simulink model "gm_transmitter"  (R2020b)
settings: Solver=FixedStepDiscrete  StartTime=0.0  StopTime=100000  RelTol=1e-3
undefined symbols (not defined in the file or in its folder): message
libraries: hdlmdlgenlib x28, simulink x10, hdlsllib x9, dspsigops x8, dspmlti4 x2, whdlio x1
(part 1 of 2)
settings Model: Creator=wardo  LastModifiedBy=wardo
settings DataIOCC: LimitDataPoints=on  SaveOutput=off  SaveTime=off
settings OptimizationCC: BlockReduction=off  ConditionallyExecuteInputs=off  DefaultParameterBehavior=Inlined  LifeSpan=inf
settings DebuggingCC: AlgebraicLoopMsg=error  InheritedTsInSrcMsg=none  SingleTaskRateTransMsg=error  AllowSymbolicDim=off  StrictBusMsg=ErrorOnBusTreatedAsVector  SFUnexpectedBacktrackingDiag=warning  SFNoUnconditionalDefaultTransitionDiag=warning  SFExecutionAtInitializationDiag=none  ArithmeticOperatorsInVariantConditions=warning
settings HardwareCC: ProdBitPerPointer=32  ProdBitPerSizeT=32  ProdBitPerPtrDiffT=32  ProdLargestAtomicFloat=None  ProdIntDivRoundTo=Undefined  ProdEndianess=Unspecified  ProdWordSize=32  ProdHWDeviceType=ASIC/FPGA->ASIC/FPGA  ProdEqTarget=off
settings SFSimCC: SimUseLocalCustomCode=off  CustomCodeUndefinedFunction=UseInterfaceOnly
settings RTWCC: RTWUseLocalCustomCode=off
settings CodeAppCC: StateflowObjectComments=on
settings GRTTargetCC: TargetLangStandard=C89/C90 (ANSI)
settings ConfigComp: CovScope=ReferencedModels  CovMetricSettings=dw  CovSaveCumulativeToWorkspaceVar=on  CovSaveSingleToWorkspaceVar=on  CovExternalEMLEnable=off  CovSFcnEnable=off

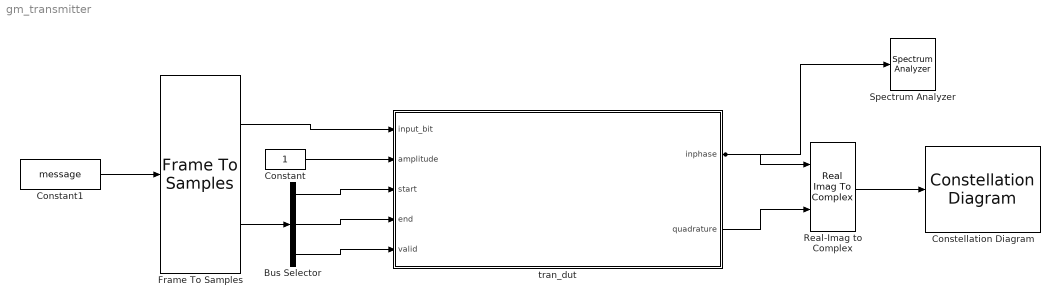
== system gm_transmitter ==
  Bus Selector : BusSelector  OutputSignals=start,end,valid
  Constant : Constant  OutDataTypeStr=uint8  SampleTime=-1
  Constant1 : Constant  Value=message  OutDataTypeStr=fixdt(0,1,0)  SampleTime=100000
  Constellation Diagram : ConstellationDiagram
  Frame To Samples : whdlio/Frame To Samples  InterSampleIdleCycles=0  InterFrameIdleCycles=0  OutputSize=1  InterleaveSamples=off
      settings: SourceProductBaseCode=LH
  Real-Imag to Complex : RealImagToComplex
  Spectrum Analyzer : SpectrumAnalyzer
  tran_dut : Subsystem
  wires:
  Bus Selector/3 -> tran_dut/5(valid)
  Bus Selector/2 -> tran_dut/4(end)
  Bus Selector/1 -> tran_dut/3(start)
  Frame To Samples/2 -> Bus Selector/1
  tran_dut/2(quadrature) -> Real-Imag to Complex/2
  tran_dut/1(inphase) -> Real-Imag to Complex/1, Spectrum Analyzer/1
  Real-Imag to Complex/1 -> Constellation Diagram/1
  Constant1/1 -> Frame To Samples/1
  Constant/1 -> tran_dut/2(amplitude)
  Frame To Samples/1 -> tran_dut/1(input_bit)

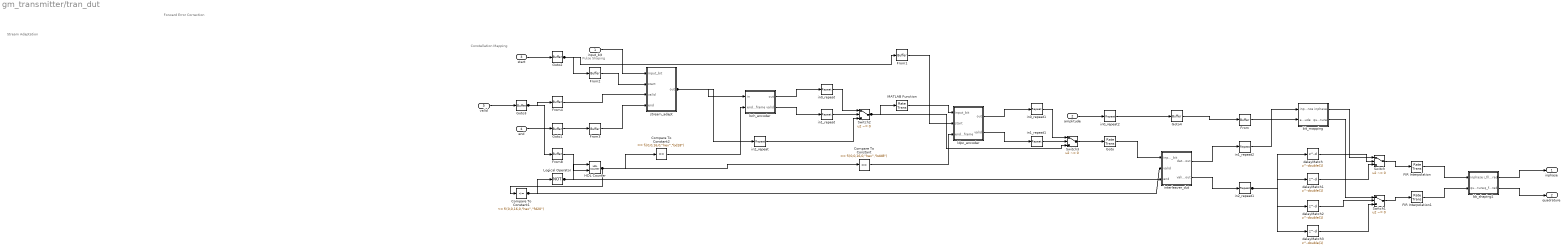
== system gm_transmitter/tran_dut ==
  note: Stream Adaptation
  note: Forward Error Correction
  note: Constellation Mapping
  note: Pulse Shaping
  input_bit : Inport  OutDataTypeStr=fixdt(0, 1, 0)  PortDimensions=1  SampleTime=2.06577425218972
  amplitude : Inport  Port=2  OutDataTypeStr=uint8  PortDimensions=1  SampleTime=2.06577425218972
  start : Inport  Port=3  OutDataTypeStr=boolean  PortDimensions=1  SampleTime=2.06577425218972
  end : Inport  Port=4  OutDataTypeStr=boolean  PortDimensions=1  SampleTime=2.06577425218972
  valid : Inport  Port=5  OutDataTypeStr=boolean  PortDimensions=1  SampleTime=2.06577425218972
  Compare To Constant : simulink/Logic and Bit Operations/Compare To Constant  relop===  const="fi(0,0,16,0,\"hex\",\"bdd8\")"  OutDataTypeStr=boolean
  Compare To Constant1 : simulink/Logic and Bit Operations/Compare To Constant  relop=<=  const="fi(0,0,16,0,\"hex\",\"fd20\")"  OutDataTypeStr=boolean
  Compare To Constant2 : simulink/Logic and Bit Operations/Compare To Constant  relop===  const="fi(0,0,16,0,\"hex\",\"bd18\")"  OutDataTypeStr=boolean
  FIR Interpolation : RateTransition  OutPortSampleTimeOpt=Multiple of input port sample time  OutPortSampleTimeMultiple=8
  FIR Interpolation1 : RateTransition  OutPortSampleTimeOpt=Multiple of input port sample time  OutPortSampleTimeMultiple=8
  From{,1..4,8} (6 alike) : hdlmdlgenlib/Buffer
      settings: SourceProductBaseCode=SL
  Goto : RateTransition  OutPortSampleTimeOpt=Multiple of input port sample time  OutPortSampleTimeMultiple=8
  Goto{1..4} (4 alike) : hdlmdlgenlib/Buffer
      settings: SourceProductBaseCode=SL
  HDL Counter : hdlsllib/Sources/HDL Counter  CountType=Count limited  CountInit=double(0)  CountStep=double(1)  CountMax=double(64800)  CountFromType=Initial value  CountFrom=double(0)  CountResetPort=on  CountLoadPort=off  CountEnbPort=on  CountDirPort=off  CountDataType=Unsigned  CountWordLen=16  CountFracLen=0  CountSampTime=2.06577425218972
  Logical Operator : Logic  Operator=NOT  Inputs=1  AllPortsSameDT=off  OutDataTypeStr=boolean  SampleTime=2.06577425218972
  MATLAB Function : RateTransition  OutPortSampleTimeOpt=Multiple of input port sample time  OutPortSampleTimeMultiple=8
  Switch : Switch  Criteria=u2 ~= 0  Threshold=double(0)  OutDataTypeStr=fixdt(1, 25, 15)  SampleTime=0.258221781523715
  Switch1 : Switch  Criteria=u2 ~= 0  Threshold=double(0)  OutDataTypeStr=fixdt(1, 25, 15)  SampleTime=0.258221781523715
  Switch2 : Switch  Criteria=u2 ~= 0  Threshold=double(0)  OutDataTypeStr=boolean  SampleTime=0.258221781523715
  Switch3 : Switch  Criteria=u2 ~= 0  Threshold=double(0)  OutDataTypeStr=boolean  SampleTime=0.258221781523715
  bb_shaping1 : Subsystem
  bch_encoder : Subsystem
  bit_mapping : Subsystem
  delayMatch{,1..3} (4 alike) : Delay  DelayLength=double(1)  InitialCondition=0  SampleTime=0.258221781523715
  in0_repeat : dspsigops/Repeat  N=double(8)  RateOptions=Allow multirate processing  ic=0  mode=Unused parameter value
  in0_repeat1 : dspsigops/Repeat  N=double(8)  RateOptions=Allow multirate processing  ic=0  mode=Unused parameter value
  in0_repeat2 : dspsigops/Repeat  N=double(8)  RateOptions=Allow multirate processing  ic=0  mode=Unused parameter value
  in1_repeat : dspsigops/Repeat  N=double(8)  RateOptions=Allow multirate processing  ic=0  mode=Unused parameter value
  in1_repeat1 : dspsigops/Repeat  N=double(8)  RateOptions=Allow multirate processing  ic=0  mode=Unused parameter value
  in1_repeat2 : dspsigops/Repeat  N=double(8)  RateOptions=Allow multirate processing  ic=0  mode=Unused parameter value
  in2_repeat : dspsigops/Repeat  N=double(8)  RateOptions=Allow multirate processing  ic=0  mode=Unused parameter value
  in2_repeat1 : dspsigops/Repeat  N=double(8)  RateOptions=Allow multirate processing  ic=0  mode=Unused parameter value
  interleaver_dut : Subsystem
  ldpc_encoder : Subsystem
  stream_adapt : Subsystem
  inphase : Outport  VectorParamsAs1DForOutWhenUnconnected=off
  quadrature : Outport  Port=2  VectorParamsAs1DForOutWhenUnconnected=off
  wires:
  input_bit/1 -> stream_adapt/1(input_bit)
  amplitude/1 -> in0_repeat2/1
  start/1 -> Goto2/1
  end/1 -> Goto1/1
  valid/1 -> Goto3/1
  From1/1 -> ldpc_encoder/2(start)
  From2/1 -> stream_adapt/2(start)
  From3/1 -> stream_adapt/4(end)
  From4/1 -> stream_adapt/3(valid)
  From8/1 -> HDL Counter/2
  HDL Counter/1 -> Compare To Constant1/1, Compare To Constant2/1, Compare To Constant/1
  bb_shaping1/1(i_filtered) -> inphase/1
  bb_shaping1/2(q_filtered) -> quadrature/1
  bch_encoder/1(out) -> in0_repeat/1
  bch_encoder/2(valid) -> in1_repeat/1
  interleaver_dut/1(data_out) -> in1_repeat2/1
  interleaver_dut/2(valid_out) -> in2_repeat1/1
  ldpc_encoder/1(out) -> in0_repeat1/1
  ldpc_encoder/2(valid) -> in1_repeat1/1
  stream_adapt/1(out) -> bch_encoder/1(in), in2_repeat/1
  Goto2/1 -> From2/1, From1/1
  Goto3/1 -> From8/1, From4/1
  Goto1/1 -> From3/1
  Compare To Constant1/1 -> interleaver_dut/2(valid), Logical Operator/1
  Logical Operator/1 -> interleaver_dut/3(end), HDL Counter/1
  Compare To Constant2/1 -> bch_encoder/2(end_of_frame)
  MATLAB Function/1 -> ldpc_encoder/1(input_bit)
  Switch2/1 -> MATLAB Function/1, Switch3/3
  Compare To Constant/1 -> ldpc_encoder/3(end_of_frame)
  Goto/1 -> interleaver_dut/1(input_bit)
  FIR Interpolation/1 -> bb_shaping1/1(inphase)
  FIR Interpolation1/1 -> bb_shaping1/2(quadrature)
  in0_repeat/1 -> Switch2/1
  in1_repeat/1 -> Switch2/2
  in2_repeat/1 -> Switch2/3
  Switch3/1 -> Goto/1
  in0_repeat1/1 -> Switch3/1
  in1_repeat1/1 -> Switch3/2
  Switch/1 -> FIR Interpolation/1
  Switch1/1 -> FIR Interpolation1/1
  in0_repeat2/1 -> Goto4/1
  in1_repeat2/1 -> bit_mapping/1(input_sequence)
  in2_repeat1/1 -> delayMatch3/1, delayMatch2/1, delayMatch1/1, delayMatch/1
  Goto4/1 -> From/1
  From/1 -> bit_mapping/2(amplitude)
  bit_mapping/1(inphase) -> Switch/1
  bit_mapping/2(quadrature) -> Switch1/1
  delayMatch/1 -> Switch/2
  delayMatch1/1 -> Switch/3
  delayMatch2/1 -> Switch1/2
  delayMatch3/1 -> Switch1/3

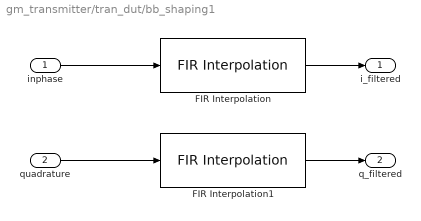
== system gm_transmitter/tran_dut/bb_shaping1 ==
  inphase : Inport  OutDataTypeStr=fixdt(1, 25, 15)  PortDimensions=1  SampleTime=2.06577425218972
  quadrature : Inport  Port=2  OutDataTypeStr=fixdt(1, 25, 15)  PortDimensions=1  SampleTime=2.06577425218972
  FIR Interpolation : dspmlti4/FIR Interpolation  FilterSource=Dialog parameters  PrivateCoeffs=0  h=[-0.00599670410156250,-0.00514221191406250,-0.00289916992187500,0.000442504882812500,0.00431823730468750,0.00794982910156250,0.0104980468750000,0.0112304687500000,0.00967407226562500,0.00578308105468750,0,-0.00680541992187500,-0.0134124755859375,-0.0184326171875000,-0.0205841064453125,-0.0189819335937500,-0.0133361816406250,-0.00410461425781250,0.00752258300781250,0.0196380615234375,0.0300140380859375,0.0363464355468750,0.0367584228515625,0.0301208496093750,0.0164794921875000,-0.00291442871093750,-0.0254821777343750,-0.0476837158203125,-0.0653228759765625,-0.0742187500000000,-0.0707244873046875,-0.0524291992187500,-0.0185852050781250,0.0296783447265625,0.0892028808593750,0.155227661132813,0.221755981445313,0.282333374023438,0.330810546875000,0.362121582031250,0.372940063476563,0.362121582031250,0.330810546875000,0.282333374023438,0.221755981445313,0.155227661132813,0.0892028808593750,0.0296783447265625,-0.0185852050781250,-0.0524291992187500,-0.0707244873046875,-0.0742187500000000,-0.0653228759765625,-0.0476837158203125,-0.0254821777343750,-0.00291442871093750,0.0164794921875000,0.0301208496093750,0.0367584228515625,0.0363464355468750,0.0300140380859375,0.0196380615234375,0.00752258300781250,-0.00410461425781250,-0.0133361816406250,-0.0189819335937500,-0.0205841064453125,-0.0184326171875000,-0.0134124755859375,-0.00680541992187500,0,0.00578308105468750,0.00967407226562500,0.0112304687500000,0.0104980468750000,0.00794982910156250,0.00431823730468750,0.000442504882812500,-0.00289916992187500,-0.00514221191406250,-0.00599670410156250]  L=8  FilterObject=FINTERP  framing=Allow multirate processing  outputBufInitCond=0  roundingMode=Floor  overflowMode=off  firstCoeffMode=Specify word length  firstCoeffWordLength=16  firstCoeffFracLength=15  firstCoeffDataTypeStr=fixdt(1,16)  firstCoeffMin=[]  firstCoeffMax=[]  firstCoeffLastDataTypeStr=fixdt(1,16)  outputDataTypeStr=Inherit: Same as accumulator  outputMin=[]  outputMax=[]  outputLastDataTypeStr=Inherit: Same as accumulator
      settings: SourceProductName=DSP System Toolbox
  FIR Interpolation1 : dspmlti4/FIR Interpolation  FilterSource=Dialog parameters  PrivateCoeffs=0  h=[-0.00599670410156250,-0.00514221191406250,-0.00289916992187500,0.000442504882812500,0.00431823730468750,0.00794982910156250,0.0104980468750000,0.0112304687500000,0.00967407226562500,0.00578308105468750,0,-0.00680541992187500,-0.0134124755859375,-0.0184326171875000,-0.0205841064453125,-0.0189819335937500,-0.0133361816406250,-0.00410461425781250,0.00752258300781250,0.0196380615234375,0.0300140380859375,0.0363464355468750,0.0367584228515625,0.0301208496093750,0.0164794921875000,-0.00291442871093750,-0.0254821777343750,-0.0476837158203125,-0.0653228759765625,-0.0742187500000000,-0.0707244873046875,-0.0524291992187500,-0.0185852050781250,0.0296783447265625,0.0892028808593750,0.155227661132813,0.221755981445313,0.282333374023438,0.330810546875000,0.362121582031250,0.372940063476563,0.362121582031250,0.330810546875000,0.282333374023438,0.221755981445313,0.155227661132813,0.0892028808593750,0.0296783447265625,-0.0185852050781250,-0.0524291992187500,-0.0707244873046875,-0.0742187500000000,-0.0653228759765625,-0.0476837158203125,-0.0254821777343750,-0.00291442871093750,0.0164794921875000,0.0301208496093750,0.0367584228515625,0.0363464355468750,0.0300140380859375,0.0196380615234375,0.00752258300781250,-0.00410461425781250,-0.0133361816406250,-0.0189819335937500,-0.0205841064453125,-0.0184326171875000,-0.0134124755859375,-0.00680541992187500,0,0.00578308105468750,0.00967407226562500,0.0112304687500000,0.0104980468750000,0.00794982910156250,0.00431823730468750,0.000442504882812500,-0.00289916992187500,-0.00514221191406250,-0.00599670410156250]  L=8  FilterObject=FINTERP  framing=Allow multirate processing  outputBufInitCond=0  roundingMode=Floor  overflowMode=off  firstCoeffMode=Specify word length  firstCoeffWordLength=16  firstCoeffFracLength=15  firstCoeffDataTypeStr=fixdt(1,16)  firstCoeffMin=[]  firstCoeffMax=[]  firstCoeffLastDataTypeStr=fixdt(1,16)  outputDataTypeStr=Inherit: Same as accumulator  outputMin=[]  outputMax=[]  outputLastDataTypeStr=Inherit: Same as accumulator
      settings: SourceProductName=DSP System Toolbox
  i_filtered : Outport  VectorParamsAs1DForOutWhenUnconnected=off
  q_filtered : Outport  Port=2  VectorParamsAs1DForOutWhenUnconnected=off
  wires:
  FIR Interpolation/1 -> i_filtered/1
  FIR Interpolation1/1 -> q_filtered/1
  inphase/1 -> FIR Interpolation/1
  quadrature/1 -> FIR Interpolation1/1

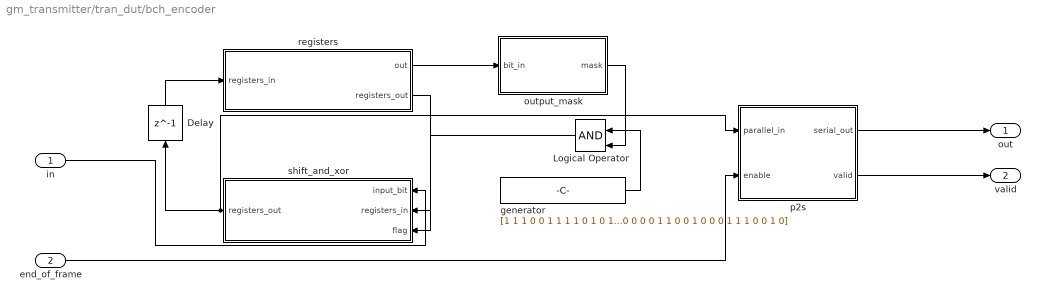
== system gm_transmitter/tran_dut/bch_encoder ==
  in : Inport  OutDataTypeStr=boolean  PortDimensions=1  SampleTime=2.06577425218972
  end_of_frame : Inport  Port=2  OutDataTypeStr=boolean  PortDimensions=1  SampleTime=2.06577425218972
  Delay : Delay  DelayLength=1
  Logical Operator : Logic  IconShape=distinctive  AllPortsSameDT=off  OutDataTypeStr=fixdt(0, 1, 0)
  generator : Constant  Value=|  OutDataTypeStr=fixdt(0, 1, 0)  SampleTime=-1
      | [1
      | 1
      | 1
      | 0
      | 0
      | 1
      | 1
      | 1
      | 1
      | 0
      | 1
      | 0
      | 1
      | 0
      | 1
      | 0
      | 0
      | 1
      | 0
      | 0
      | 0
      | 0
      | 0
      | 0
      | 0
      | 1
      | 1
      | 0
      | 0
      | 1
      | 1
      | 0
      | 1
      | 1
      | 1
      | 0
      | 1
      | 1
      | 1
      | 1
      | 1
      | 0
      | 1
      | 0
      | 0
      | 0
      | 0
      | 1
      | 1
      | 1
      | 1
      | 0
      | 0
      | 0
      | 1
      | 0
      | 1
      | 1
      | 0
      | 0
      | 0
      | 0
      | 0
      | 0
      | 1
      | 0
      | 0
      | 1
      | 0
      | 0
      | 0
      | 1
      | 0
      | 0
      | 0
      | 1
      | 0
      | 0
      | 0
      | 0
      | 1
      | 0
      | 1
      | 0
      | 1
      | 1
      | 0
      | 0
      | 0
      | 0
      | 1
      | 1
      | 1
      | 0
      | 1
      | 1
      | 0
      | 0
      | 0
      | 1
      | 1
      | 0
      | 1
      | 1
      | 0
      | 0
      | 1
      | 1
      | 0
      | 1
      | 0
      | 0
      | 1
      | 1
      | 1
      | 1
      | 0
      | 0
      | 1
      | 1
      | 0
      | 0
      | 0
      | 0
      | 1
      | 0
      | 1
      | 0
      | 0
      | 0
      | 1
      | 1
      | 1
      | 0
      | 0
      | 0
      | 1
      | 0
      | 0
      | 0
      | 1
      | 0
      | 1
      | 0
      | 0
      | 0
      | 1
      | 1
      | 1
      | 0
      | 1
      | 0
      | 0
      | 0
      | 1
      | 0
      | 0
      | 0
      | 0
      | 1
      | 1
      | 1
      | 0
      | 0
      | 0
      | 0
      | 0
      | 1
      | 0
      | 1
      | 1
      | 1
      | 0
      | 0
      | 0
      | 0
      | 0
      | 1
      | 1
      | 0
      | 0
      | 1
      | 0
      | 0
      | 0
      | 1
      | 1
      | 1
      | 0
      | 0
      | 1
      | 0]
  output_mask : Subsystem
  p2s : Subsystem
  registers : Subsystem
  shift_and_xor : Subsystem
  out : Outport  VectorParamsAs1DForOutWhenUnconnected=off
  valid : Outport  Port=2  VectorParamsAs1DForOutWhenUnconnected=off
  wires:
  generator/1 -> Logical Operator/1
  p2s/1(serial_out) -> out/1
  p2s/2(valid) -> valid/1
  shift_and_xor/1(registers_out) -> p2s/1(parallel_in), Delay/1
  in/1 -> shift_and_xor/1(input_bit)
  end_of_frame/1 -> p2s/2(enable)
  Logical Operator/1 -> shift_and_xor/3(flag)
  output_mask/1(mask) -> Logical Operator/2
  Delay/1 -> registers/1(registers_in)
  registers/1(out) -> output_mask/1(bit_in)
  registers/2(registers_out) -> shift_and_xor/2(registers_in)

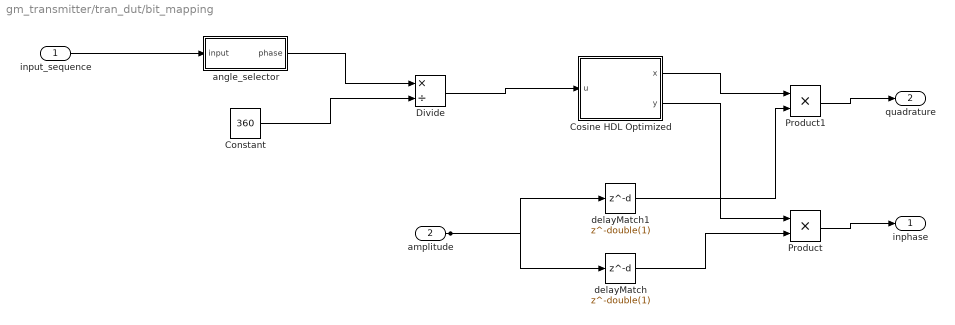
== system gm_transmitter/tran_dut/bit_mapping ==
  input_sequence : Inport  OutDataTypeStr=fixdt(0, 3, 0)  PortDimensions=1  SampleTime=0.258221781523715
  amplitude : Inport  Port=2  OutDataTypeStr=uint8  PortDimensions=1  SampleTime=0.258221781523715
  Constant : Constant  Value=360  OutDataTypeStr=fixdt(0, 9, 0)  SampleTime=0.258221781523715
  Cosine HDL Optimized : Subsystem  mask(Sine and Cosine HDL optimized block){OutputFormula=sin(2*pi*u) and cos(2*pi*u), NumDataPoints=double(32), TableDataTypeStr=fixdt(1,16,15), SimulateLUTROMDelay=off}
      mask prompts: OutputFormula "Simulink:masks:OutputFormula_MP"; NumDataPoints "HDLShared:hdlshared:CosineHDL_Npts"; TableDataTypeStr "Simulink:blkprm_prompts:TABLE_UNIFIEDDATATYPE"; SimulateLUTROMDelay "HDLShared:hdlshared:CosineHDL_Map2RAM"
      mask help: Sine and Cosine HDL optimized block using quarter wave symmetry, and HDL friendly settings.
      mask Help: helpview([docroot '/hdlcoder/helptargets.map'],'SineAndCosineHDL_Optimized');
      mask TypeOptions OutputFormula: sin(2*pi*u) | cos(2*pi*u) | exp(j*2*pi*u) | sin(2*pi*u) and cos(2*pi*u)
      mask Display:
      | port_label('input',1,'u')
      | port_label('output',1,'sin(2*pi*u)')
      | port_label('output',2,'cos(2*pi*u)')
      | xpos = 0.35;
      | yoffset = 0.5;
      | if ( SimulateLUTROMDelay )
      |   text(xpos,yoffset,'HDL (Z^{-1})','texmode','on')
      | else
      |    text(xpos,yoffset,'HDL')
      | end
  Divide : Product  Inputs=*/  OutDataTypeStr=fixdt(1, 16, 14)  RndMeth=Zero  SaturateOnIntegerOverflow=on  SampleTime=0.258221781523715
  Product : Product  Inputs=**  OutDataTypeStr=fixdt(1, 25, 15)  SampleTime=0.258221781523715
  Product1 : Product  Inputs=**  OutDataTypeStr=fixdt(1, 25, 15)  SampleTime=0.258221781523715
  angle_selector : Subsystem
  delayMatch : Delay  DelayLength=double(1)  InitialCondition=0  SampleTime=0.258221781523715
  delayMatch1 : Delay  DelayLength=double(1)  InitialCondition=0  SampleTime=0.258221781523715
  inphase : Outport  VectorParamsAs1DForOutWhenUnconnected=off
  quadrature : Outport  Port=2  VectorParamsAs1DForOutWhenUnconnected=off
  wires:
  delayMatch/1 -> Product/2
  Constant/1 -> Divide/2
  Cosine HDL Optimized/1(x) -> Product1/1
  Cosine HDL Optimized/2(y) -> Product/1
  Divide/1 -> Cosine HDL Optimized/1(u)
  Product/1 -> inphase/1
  Product1/1 -> quadrature/1
  angle_selector/1(phase) -> Divide/1
  delayMatch1/1 -> Product1/2
  input_sequence/1 -> angle_selector/1(input)
  amplitude/1 -> delayMatch1/1, delayMatch/1

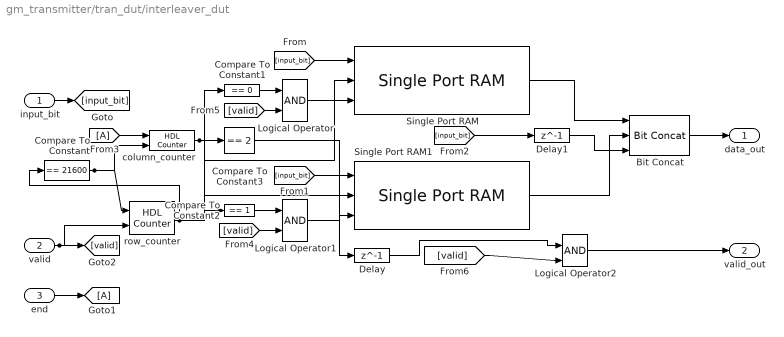
== system gm_transmitter/tran_dut/interleaver_dut ==
  input_bit : Inport  OutDataTypeStr=boolean  PortDimensions=1  SampleTime=2.06577425218972
  valid : Inport  Port=2  OutDataTypeStr=boolean  PortDimensions=1  SampleTime=2.06577425218972
  end : Inport  Port=3  OutDataTypeStr=boolean  PortDimensions=1  SampleTime=2.06577425218972
  Bit Concat : hdlsllib/Logic and Bit Operations/Bit Concat  numInputs=3
  Compare To Constant : simulink/Logic and Bit Operations/Compare To Constant  relop===  const=21600  OutDataTypeStr=boolean
  Compare To Constant1 : simulink/Logic and Bit Operations/Compare To Constant  relop===  const=0  OutDataTypeStr=boolean
  Compare To Constant2 : simulink/Logic and Bit Operations/Compare To Constant  relop===  const=1  OutDataTypeStr=boolean
  Compare To Constant3 : simulink/Logic and Bit Operations/Compare To Constant  relop===  const=2  OutDataTypeStr=boolean
  Delay : Delay  DelayLength=1
  Delay1 : Delay  DelayLength=1
  Logical Operator : Logic  IconShape=distinctive  AllPortsSameDT=off  OutDataTypeStr=boolean
  Logical Operator1 : Logic  IconShape=distinctive  AllPortsSameDT=off  OutDataTypeStr=boolean
  Logical Operator2 : Logic  IconShape=distinctive  AllPortsSameDT=off  OutDataTypeStr=boolean
  Single Port RAM : hdlsllib/HDL RAMs/Single Port RAM  ram_size=15  dout_type=New data
      settings: SourceProductBaseCode=SL
  Single Port RAM1 : hdlsllib/HDL RAMs/Single Port RAM  ram_size=15  dout_type=New data
      settings: SourceProductBaseCode=SL
  column_counter : hdlsllib/Sources/HDL Counter  CountType=Count limited  CountInit=0  CountStep=1  CountMax=2  CountFromType=Initial value  CountFrom=0  CountResetPort=on  CountLoadPort=off  CountEnbPort=on  CountDirPort=off  CountDataType=Unsigned  CountWordLen=3  CountFracLen=0  CountSampTime=1
  row_counter : hdlsllib/Sources/HDL Counter  CountType=Count limited  CountInit=1  CountStep=1  CountMax=21600  CountFromType=Initial value  CountFrom=1  CountResetPort=on  CountLoadPort=off  CountEnbPort=on  CountDirPort=off  CountDataType=Unsigned  CountWordLen=15  CountFracLen=0  CountSampTime=1
  data_out : Outport  VectorParamsAs1DForOutWhenUnconnected=off
  valid_out : Outport  Port=2  VectorParamsAs1DForOutWhenUnconnected=off
  wires:
  Bit Concat/1 -> data_out/1
  Compare To Constant/1 -> column_counter/2, row_counter/1
  Compare To Constant1/1 -> Logical Operator/1
  Compare To Constant2/1 -> Logical Operator1/1
  Compare To Constant3/1 -> Delay/1
  Delay/1 -> Logical Operator2/1
  Delay1/1 -> Bit Concat/3
  [input_bit] -> Single Port RAM/1
  [input_bit] -> Single Port RAM1/1
  [input_bit] -> Delay1/1
  [A] -> column_counter/1
  [valid] -> Logical Operator1/2
  [valid] -> Logical Operator/2
  [valid] -> Logical Operator2/2
  Logical Operator/1 -> Single Port RAM/3
  Logical Operator1/1 -> Single Port RAM1/3
  Logical Operator2/1 -> valid_out/1
  Single Port RAM/1 -> Bit Concat/1
  Single Port RAM1/1 -> Bit Concat/2
  column_counter/1 -> Compare To Constant3/1, Compare To Constant2/1, Compare To Constant1/1
  row_counter/1 -> Compare To Constant/1, Single Port RAM/2, Single Port RAM1/2
  input_bit/1 -> [input_bit]
  valid/1 -> [valid], row_counter/2
  end/1 -> [A]

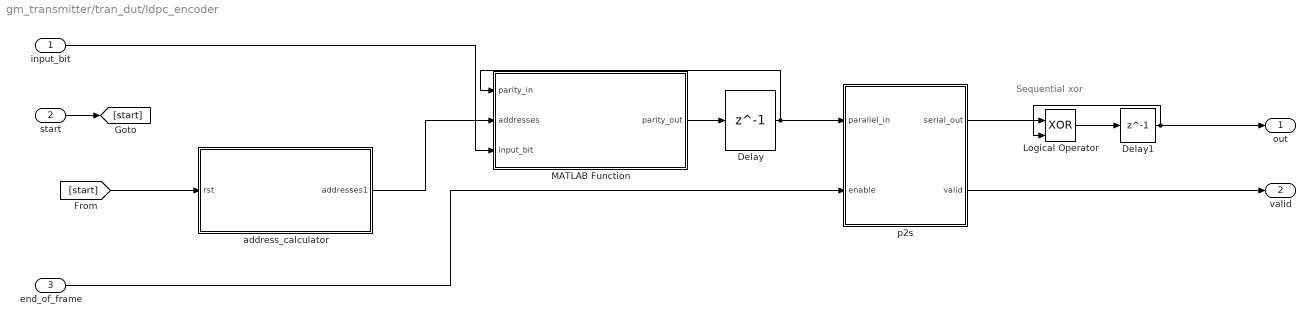
== system gm_transmitter/tran_dut/ldpc_encoder ==
  note: Sequential xor
  input_bit : Inport  OutDataTypeStr=boolean  PortDimensions=1  SampleTime=2.06577425218972
  start : Inport  Port=2  OutDataTypeStr=boolean  PortDimensions=1  SampleTime=2.06577425218972
  end_of_frame : Inport  Port=3  OutDataTypeStr=boolean  PortDimensions=1  SampleTime=2.06577425218972
  Delay : Delay  DelayLength=1  InitialCondition=[zeros(16200, 1); 1]
  Delay1 : Delay  DelayLength=1
  Logical Operator : Logic  Operator=XOR  IconShape=distinctive  AllPortsSameDT=off  OutDataTypeStr=fixdt(0,1, 0)
  MATLAB Function : Subsystem
  address_calculator : Subsystem
  p2s : Subsystem
  out : Outport  VectorParamsAs1DForOutWhenUnconnected=off
  valid : Outport  Port=2  VectorParamsAs1DForOutWhenUnconnected=off
  wires:
  Delay/1 -> p2s/1(parallel_in), MATLAB Function/1(parity_in)
  Delay1/1 -> out/1, Logical Operator/2
  [start] -> address_calculator/1(rst)
  address_calculator/1(addresses1) -> MATLAB Function/2(addresses)
  p2s/1(serial_out) -> Logical Operator/1
  p2s/2(valid) -> valid/1
  input_bit/1 -> MATLAB Function/3(input_bit)
  start/1 -> [start]
  end_of_frame/1 -> p2s/2(enable)
  MATLAB Function/1(parity_out) -> Delay/1
  Logical Operator/1 -> Delay1/1

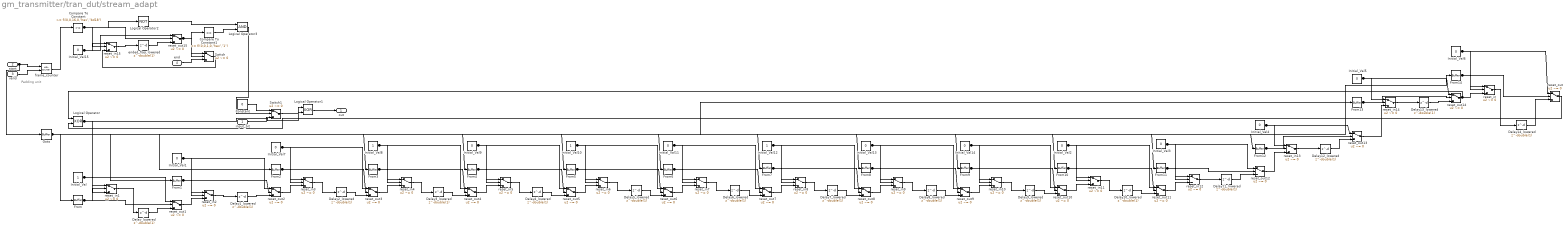
== system gm_transmitter/tran_dut/stream_adapt ==
  note: Padding unit
  input_bit : Inport  OutDataTypeStr=fixdt(0, 1, 0)  PortDimensions=1  SampleTime=2.06577425218972
  start : Inport  Port=2  OutDataTypeStr=boolean  PortDimensions=1  SampleTime=2.06577425218972
  valid : Inport  Port=3  OutDataTypeStr=boolean  PortDimensions=1  SampleTime=2.06577425218972
  end : Inport  Port=4  OutDataTypeStr=boolean  PortDimensions=1  SampleTime=2.06577425218972
  Compare To Constant : simulink/Logic and Bit Operations/Compare To Constant  relop=>=  const="fi(0,0,16,0,\"hex\",\"bd18\")"  OutDataTypeStr=boolean
  Compare To Constant1 : simulink/Logic and Bit Operations/Compare To Constant  relop===  const="fi(0,0,1,0,\"hex\",\"1\")"  OutDataTypeStr=boolean
  Constant : Constant  Value=0  OutDataTypeStr=fixdt(0, 1, 1000)  SampleTime=2.06577425218972
  Delay10_lowered : Delay  DelayLength=double(1)  InitialCondition=0  SampleTime=2.06577425218972
  Delay11_lowered : Delay  DelayLength=double(1)  InitialCondition=0  SampleTime=2.06577425218972
  Delay12_lowered : Delay  DelayLength=double(1)  InitialCondition=0  SampleTime=2.06577425218972
  Delay13_lowered : Delay  DelayLength=double(1)  InitialCondition=0  SampleTime=2.06577425218972
  Delay14_lowered : Delay  DelayLength=double(1)  InitialCondition=0  SampleTime=2.06577425218972
  Delay1_lowered : Delay  DelayLength=double(1)  InitialCondition=0  SampleTime=2.06577425218972
  Delay2_lowered : Delay  DelayLength=double(1)  InitialCondition=0  SampleTime=2.06577425218972
  Delay3_lowered : Delay  DelayLength=double(1)  InitialCondition=1  SampleTime=2.06577425218972
  Delay4_lowered : Delay  DelayLength=double(1)  InitialCondition=0  SampleTime=2.06577425218972
  Delay5_lowered : Delay  DelayLength=double(1)  InitialCondition=1  SampleTime=2.06577425218972
  Delay6_lowered : Delay  DelayLength=double(1)  InitialCondition=0  SampleTime=2.06577425218972
  Delay7_lowered : Delay  DelayLength=double(1)  InitialCondition=1  SampleTime=2.06577425218972
  Delay8_lowered : Delay  DelayLength=double(1)  InitialCondition=0  SampleTime=2.06577425218972
  Delay9_lowered : Delay  DelayLength=double(1)  InitialCondition=0  SampleTime=2.06577425218972
  Delay_lowered : Delay  DelayLength=double(1)  InitialCondition=1  SampleTime=2.06577425218972
  From{,1..14} (15 alike) : hdlmdlgenlib/Buffer
      settings: SourceProductBaseCode=SL
  Goto : hdlmdlgenlib/Buffer
      settings: SourceProductBaseCode=SL
  Initial_Val{,8,10,12} (4 alike) : Constant  OutDataTypeStr=boolean  SampleTime=2.06577425218972
  Initial_Val{1..7,9,11,13..15} (12 alike) : Constant  Value=0  OutDataTypeStr=boolean  SampleTime=2.06577425218972
  Logical Operator : Logic  Operator=XOR  AllPortsSameDT=off  OutDataTypeStr=boolean  SampleTime=2.06577425218972
  Logical Operator1 : Logic  Operator=XOR  AllPortsSameDT=off  OutDataTypeStr=boolean  SampleTime=2.06577425218972
  Logical Operator2 : Logic  Operator=NOT  Inputs=1  AllPortsSameDT=off  OutDataTypeStr=boolean  SampleTime=2.06577425218972
  Logical Operator3 : Logic  AllPortsSameDT=off  OutDataTypeStr=boolean  SampleTime=2.06577425218972
  Switch : Switch  Criteria=u2 ~= 0  Threshold=double(0)  OutDataTypeStr=boolean  SampleTime=2.06577425218972
  Switch1 : Switch  Criteria=u2 ~= 0  Threshold=double(0)  OutDataTypeStr=fixdt(0, 1, 0)  SampleTime=2.06577425218972
  ended_flag_lowered : Delay  DelayLength=double(1)  InitialCondition=0  SampleTime=2.06577425218972
  frame_counter : hdlsllib/Sources/HDL Counter  CountType=Count limited  CountInit=double(0)  CountStep=double(1)  CountMax=double(48408)  CountFromType=Initial value  CountFrom=double(0)  CountResetPort=on  CountLoadPort=off  CountEnbPort=on  CountDirPort=off  CountDataType=Unsigned  CountWordLen=16  CountFracLen=0  CountSampTime=2.06577425218972
  reset_in{,1..15} (16 alike) : Switch  Criteria=u2 ~= 0  Threshold=double(0)  OutDataTypeStr=boolean  SampleTime=2.06577425218972
  reset_out{,1..15} (16 alike) : Switch  Criteria=u2 ~= 0  Threshold=double(0)  OutDataTypeStr=boolean  SampleTime=2.06577425218972
  out : Outport  VectorParamsAs1DForOutWhenUnconnected=off
  wires:
  Compare To Constant/1 -> Logical Operator2/1, reset_out15/2, reset_in15/2
  Compare To Constant1/1 -> Logical Operator3/2
  Constant/1 -> Switch1/1
  From/1 -> reset_out1/2, reset_in1/2
  From1/1 -> reset_out2/2, reset_in2/2
  From10/1 -> reset_out11/2, reset_in11/2
  From11/1 -> reset_out12/2, reset_in12/2
  From12/1 -> reset_out13/2, reset_in13/2
  From13/1 -> reset_out14/2, reset_in14/2
  From14/1 -> reset_out/2, reset_in/2
  From2/1 -> reset_out3/2, reset_in3/2
  From3/1 -> reset_out4/2, reset_in4/2
  From4/1 -> reset_out5/2, reset_in5/2
  From5/1 -> reset_out6/2, reset_in6/2
  From6/1 -> reset_out7/2, reset_in7/2
  From7/1 -> reset_out8/2, reset_in8/2
  From8/1 -> reset_out9/2, reset_in9/2
  From9/1 -> reset_out10/2, reset_in10/2
  Logical Operator/1 -> Logical Operator1/1, reset_in1/3
  Logical Operator1/1 -> out/1
  Logical Operator2/1 -> Logical Operator3/1
  Logical Operator3/1 -> Switch1/2
  Switch1/1 -> Logical Operator1/2
  reset_out15/1 -> Compare To Constant1/1, Switch/2, Switch/1
  frame_counter/1 -> Compare To Constant/1
  Goto/1 -> From9/1, From8/1, From7/1, From6/1, From5/1, From4/1, From3/1, From2/1, From14/1, From13/1, From12/1, From11/1, From10/1, From1/1, From/1
  Initial_Val/1 -> reset_out1/1, reset_in1/1
  Initial_Val1/1 -> reset_out2/1, reset_in2/1
  Initial_Val2/1 -> reset_out11/1, reset_in11/1
  Initial_Val3/1 -> reset_out12/1, reset_in12/1
  Initial_Val4/1 -> reset_out13/1, reset_in13/1
  Initial_Val5/1 -> reset_out14/1, reset_in14/1
  Initial_Val6/1 -> reset_out/1, reset_in/1
  Initial_Val7/1 -> reset_out3/1, reset_in3/1
  Initial_Val8/1 -> reset_out4/1, reset_in4/1
  Initial_Val9/1 -> reset_out5/1, reset_in5/1
  Initial_Val10/1 -> reset_out6/1, reset_in6/1
  Initial_Val11/1 -> reset_out7/1, reset_in7/1
  Initial_Val12/1 -> reset_out8/1, reset_in8/1
  Initial_Val13/1 -> reset_out9/1, reset_in9/1
  Initial_Val14/1 -> reset_out10/1, reset_in10/1
  Initial_Val15/1 -> reset_out15/1, reset_in15/1
  input_bit/1 -> Switch1/3
  start/1 -> frame_counter/1, Goto/1
  valid/1 -> frame_counter/2
  end/1 -> Switch/3
  reset_in/1 -> Delay14_lowered/1
  Delay14_lowered/1 -> reset_out/3
  reset_out/1 -> Logical Operator/2
  reset_in1/1 -> Delay_lowered/1
  Delay_lowered/1 -> reset_out1/3
  reset_out1/1 -> reset_in2/3
  reset_in2/1 -> Delay1_lowered/1
  Delay1_lowered/1 -> reset_out2/3
  reset_out2/1 -> reset_in3/3
  reset_in3/1 -> Delay2_lowered/1
  Delay2_lowered/1 -> reset_out3/3
  reset_out3/1 -> reset_in4/3
  reset_in4/1 -> Delay3_lowered/1
  Delay3_lowered/1 -> reset_out4/3
  reset_out4/1 -> reset_in5/3
  reset_in5/1 -> Delay4_lowered/1
  Delay4_lowered/1 -> reset_out5/3
  reset_out5/1 -> reset_in6/3
  reset_in6/1 -> Delay5_lowered/1
  Delay5_lowered/1 -> reset_out6/3
  reset_out6/1 -> reset_in7/3
  reset_in7/1 -> Delay6_lowered/1
  Delay6_lowered/1 -> reset_out7/3
  reset_out7/1 -> reset_in8/3
  reset_in8/1 -> Delay7_lowered/1
  Delay7_lowered/1 -> reset_out8/3
  reset_out8/1 -> reset_in9/3
  reset_in9/1 -> Delay8_lowered/1
  Delay8_lowered/1 -> reset_out9/3
  reset_out9/1 -> reset_in10/3
  reset_in10/1 -> Delay9_lowered/1
  Delay9_lowered/1 -> reset_out10/3
  reset_out10/1 -> reset_in11/3
  reset_in11/1 -> Delay10_lowered/1
  Delay10_lowered/1 -> reset_out11/3
  reset_out11/1 -> reset_in12/3
  reset_in12/1 -> Delay11_lowered/1
  Delay11_lowered/1 -> reset_out12/3
  reset_out12/1 -> reset_in13/3
  reset_in13/1 -> Delay12_lowered/1
  Delay12_lowered/1 -> reset_out13/3
  reset_out13/1 -> reset_in14/3
  reset_in14/1 -> Delay13_lowered/1
  Delay13_lowered/1 -> reset_out14/3
  reset_out14/1 -> Logical Operator/1, reset_in/3
  Switch/1 -> reset_in15/3
  reset_in15/1 -> ended_flag_lowered/1
  ended_flag_lowered/1 -> reset_out15/3

== system gm_transmitter/tran_dut/bch_encoder/output_mask ==
  bit_in : Inport  OutDataTypeStr=fixdt(0, 1, 0)  PortDimensions=1  SampleTime=2.06577425218972
  output_mask : MATLAB Function  TreatAsAtomicUnit=on
  mask : Outport  VectorParamsAs1DForOutWhenUnconnected=off
  wires:
  bit_in/1 -> output_mask/1(bit_in)
  output_mask/1(mask) -> mask/1

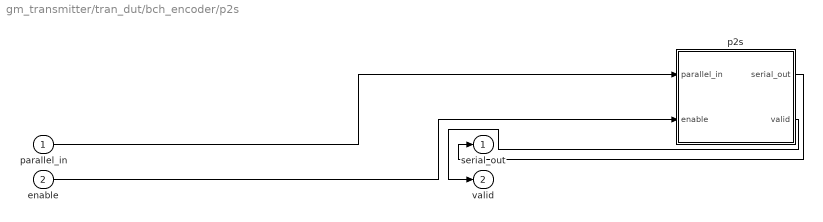
== system gm_transmitter/tran_dut/bch_encoder/p2s ==
  parallel_in : Inport  OutDataTypeStr=fixdt(0, 1, 0)  PortDimensions=[192]  SampleTime=2.06577425218972
  enable : Inport  Port=2  OutDataTypeStr=boolean  PortDimensions=1  SampleTime=2.06577425218972
  p2s : MATLAB Function  TreatAsAtomicUnit=on  mask{input_length=192}
  serial_out : Outport  VectorParamsAs1DForOutWhenUnconnected=off
  valid : Outport  Port=2
  wires:
  p2s/1(serial_out) -> serial_out/1
  p2s/2(valid) -> valid/1
  parallel_in/1 -> p2s/1(parallel_in)
  enable/1 -> p2s/2(enable)

== system gm_transmitter/tran_dut/bch_encoder/registers ==
  registers_in : Inport  OutDataTypeStr=fixdt(0, 1, 0)  PortDimensions=[192]  SampleTime=2.06577425218972
  registers : MATLAB Function  TreatAsAtomicUnit=on
  out : Outport  VectorParamsAs1DForOutWhenUnconnected=off
  registers_out : Outport  Port=2
  wires:
  registers_in/1 -> registers/1(registers_in)
  registers/1(out) -> out/1
  registers/2(registers_out) -> registers_out/1

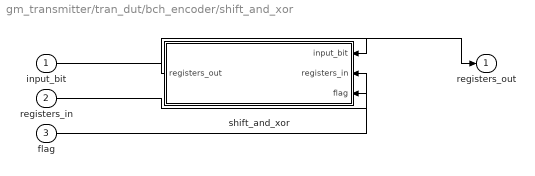
== system gm_transmitter/tran_dut/bch_encoder/shift_and_xor ==
  input_bit : Inport  OutDataTypeStr=boolean  PortDimensions=1  SampleTime=2.06577425218972
  registers_in : Inport  Port=2  OutDataTypeStr=fixdt(0, 1, 0)  PortDimensions=[192]  SampleTime=2.06577425218972
  flag : Inport  Port=3  OutDataTypeStr=fixdt(0, 1, 0)  PortDimensions=[192]  SampleTime=2.06577425218972
  shift_and_xor : MATLAB Function  TreatAsAtomicUnit=on
  registers_out : Outport  VectorParamsAs1DForOutWhenUnconnected=off
  wires:
  input_bit/1 -> shift_and_xor/1(input_bit)
  registers_in/1 -> shift_and_xor/2(registers_in)
  flag/1 -> shift_and_xor/3(flag)
  shift_and_xor/1(registers_out) -> registers_out/1

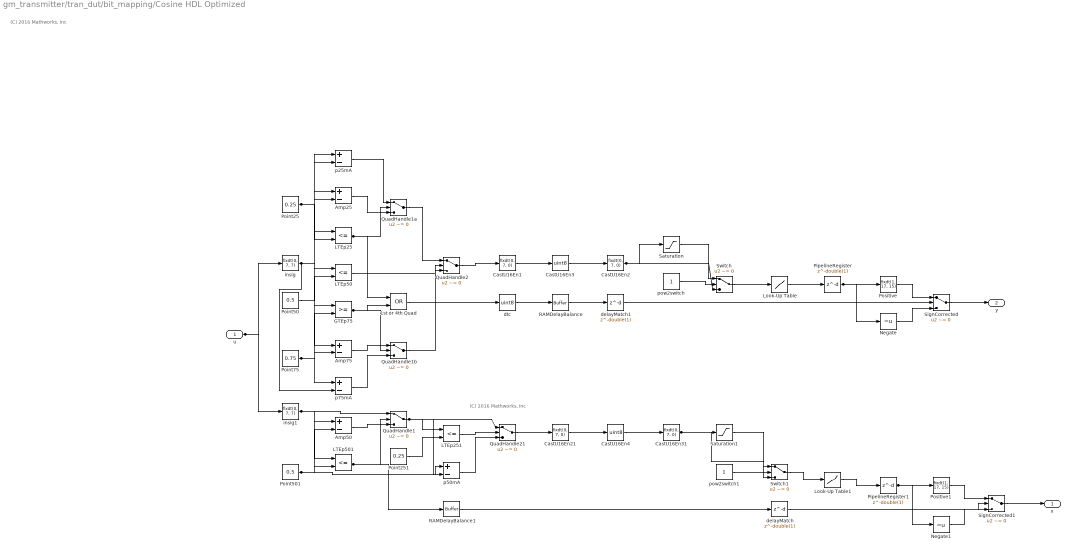
== system gm_transmitter/tran_dut/bit_mapping/Cosine HDL Optimized ==
  note: (C) 2016 Mathworks, Inc
  note: (C) 2016 Mathworks, Inc
  u : Inport  OutDataTypeStr=fixdt(1, 16, 14)  SampleTime=0.258221781523715
  1st or 4th Quad : Logic  Operator=OR  AllPortsSameDT=off  OutDataTypeStr=boolean  SampleTime=0.258221781523715
  Amp25 : Sum  Inputs=+-  AccumDataTypeStr=fixdt(1, 18, 17)  OutDataTypeStr=fixdt(1, 18, 17)  SampleTime=0.258221781523715
  Amp50 : Sum  Inputs=+-  AccumDataTypeStr=fixdt(1, 18, 17)  OutDataTypeStr=fixdt(1, 18, 17)  SampleTime=0.258221781523715
  Amp75 : Sum  Inputs=+-  AccumDataTypeStr=fixdt(1, 18, 17)  OutDataTypeStr=fixdt(1, 18, 17)  SampleTime=0.258221781523715
  CastU16En1 : DataTypeConversion  OutDataTypeStr=fixdt(0, 7, 0)  ConvertRealWorld=Stored Integer (SI)  SampleTime=0.258221781523715
  CastU16En2 : DataTypeConversion  OutDataTypeStr=fixdt(0, 7, 0)  ConvertRealWorld=Stored Integer (SI)  SampleTime=0.258221781523715  SaturateOnIntegerOverflow=on
  CastU16En21 : DataTypeConversion  OutDataTypeStr=fixdt(0, 7, 0)  ConvertRealWorld=Stored Integer (SI)  SampleTime=0.258221781523715
  CastU16En3 : DataTypeConversion  OutDataTypeStr=uint8  SampleTime=0.258221781523715
  CastU16En31 : DataTypeConversion  OutDataTypeStr=fixdt(0, 7, 0)  ConvertRealWorld=Stored Integer (SI)  SampleTime=0.258221781523715  SaturateOnIntegerOverflow=on
  CastU16En4 : DataTypeConversion  OutDataTypeStr=uint8  SampleTime=0.258221781523715
  GTEp75 : RelationalOperator  OutDataTypeStr=boolean  SampleTime=0.258221781523715  RndMeth=Nearest
  LTEp{25,50,251,501} (4 alike) : RelationalOperator  Operator=<=  OutDataTypeStr=boolean  SampleTime=0.258221781523715  RndMeth=Nearest
  Look-Up Table : Lookup_n-D  NumberOfTableDimensions=1  BreakpointsForDimension1="fi(\"numerictype\",numerictype(0,7,0),\"fimath\",fimath(\"RoundingMethod\", \"Floor\",\"OverflowAction\", \"Wrap\",\"ProductMode\",\"FullPrecision\",\"SumMode\",\"FullPrecision\"),\"Value\",\"[0 1 2 3 4 5 6 7 8 9 10 11 12 13 14 15 16 17 18 19 20 21 22 23 24 25 26 27 28 29 30 31]\")"  Table="reshape(fi(\"numerictype\",numerictype(1,17,15),\"fimath\",fimath(\"RoundingMethod\", \"Floor\",\"OverflowAction\", \"Wrap\",\"ProductMode\",\"FullPrecision\",\"SumMode\",\"FullPrecision\"),\"Value\",\"[0;0.0506591796875;0.101165771484375;0.15142822265625;0.2012939453125;0.250640869140625;0.29937744140625;0.3472900390625;0.39434814453125;0.440399169921875;0.48529052734375;0.528961181640625;0.571258544921875;0.612091064453125;0.6513671875;0.68896484375;0.72479248046875;0.758758544921875;0.790771484375;0.820770263671875;0.8486328125;0.874359130859375;0.897796630859375;0.9189453125;0.937744140625;0.954132080078125;0.96807861328125;0.979522705078125;0.98846435546875;0.994873046875;0.99871826171875;1]\"), [1  32])"  InterpMethod=Flat  ExtrapMethod=Clip  DiagnosticForOutOfRangeInput=Error  SampleTime=0.258221781523715  OutDataTypeStr=fixdt(1, 17, 15)  InputSameDT=on
  Look-Up Table1 : Lookup_n-D  NumberOfTableDimensions=1  BreakpointsForDimension1="fi(\"numerictype\",numerictype(0,7,0),\"fimath\",fimath(\"RoundingMethod\", \"Floor\",\"OverflowAction\", \"Wrap\",\"ProductMode\",\"FullPrecision\",\"SumMode\",\"FullPrecision\"),\"Value\",\"[0 1 2 3 4 5 6 7 8 9 10 11 12 13 14 15 16 17 18 19 20 21 22 23 24 25 26 27 28 29 30 31]\")"  Table="reshape(fi(\"numerictype\",numerictype(1,17,15),\"fimath\",fimath(\"RoundingMethod\", \"Floor\",\"OverflowAction\", \"Wrap\",\"ProductMode\",\"FullPrecision\",\"SumMode\",\"FullPrecision\"),\"Value\",\"[0;0.0506591796875;0.101165771484375;0.15142822265625;0.2012939453125;0.250640869140625;0.29937744140625;0.3472900390625;0.39434814453125;0.440399169921875;0.48529052734375;0.528961181640625;0.571258544921875;0.612091064453125;0.6513671875;0.68896484375;0.72479248046875;0.758758544921875;0.790771484375;0.820770263671875;0.8486328125;0.874359130859375;0.897796630859375;0.9189453125;0.937744140625;0.954132080078125;0.96807861328125;0.979522705078125;0.98846435546875;0.994873046875;0.99871826171875;1]\"), [1  32])"  InterpMethod=Flat  ExtrapMethod=Clip  DiagnosticForOutOfRangeInput=Error  SampleTime=0.258221781523715  OutDataTypeStr=fixdt(1, 17, 15)  InputSameDT=on
  Negate : UnaryMinus  SampleTime=0.258221781523715
  Negate1 : UnaryMinus  SampleTime=0.258221781523715
  PipelineRegister : Delay  DelayLength=double(1)  InitialCondition=0  SampleTime=0.258221781523715
  PipelineRegister1 : Delay  DelayLength=double(1)  InitialCondition=0  SampleTime=0.258221781523715
  Point25 : Constant  Value=0.25  OutDataTypeStr=fixdt(0, 17, 17)  SampleTime=0.258221781523715
  Point251 : Constant  Value=0.25  OutDataTypeStr=fixdt(0, 17, 17)  SampleTime=0.258221781523715
  Point50 : Constant  Value=0.5  OutDataTypeStr=fixdt(0, 17, 17)  SampleTime=0.258221781523715
  Point501 : Constant  Value=0.5  OutDataTypeStr=fixdt(0, 17, 17)  SampleTime=0.258221781523715
  Point75 : Constant  Value=0.75  OutDataTypeStr=fixdt(0, 17, 17)  SampleTime=0.258221781523715
  Positive : DataTypeConversion  OutDataTypeStr=fixdt(1, 17, 15)  SampleTime=0.258221781523715
  Positive1 : DataTypeConversion  OutDataTypeStr=fixdt(1, 17, 15)  SampleTime=0.258221781523715
  QuadHandle1 : Switch  Criteria=u2 ~= 0  Threshold=double(0)  OutDataTypeStr=fixdt(1, 18, 17)  SampleTime=0.258221781523715
  QuadHandle1a : Switch  Criteria=u2 ~= 0  Threshold=double(0)  OutDataTypeStr=fixdt(1, 18, 17)  SampleTime=0.258221781523715
  QuadHandle1b : Switch  Criteria=u2 ~= 0  Threshold=double(0)  OutDataTypeStr=fixdt(1, 18, 17)  SampleTime=0.258221781523715
  QuadHandle2 : Switch  Criteria=u2 ~= 0  Threshold=double(0)  OutDataTypeStr=fixdt(0, 7, 7)  SampleTime=0.258221781523715  SaturateOnIntegerOverflow=on
  QuadHandle21 : Switch  Criteria=u2 ~= 0  Threshold=double(0)  OutDataTypeStr=fixdt(0, 7, 7)  SampleTime=0.258221781523715
  RAMDelayBalance : hdlmdlgenlib/Buffer
      settings: SourceProductBaseCode=SL
  RAMDelayBalance1 : hdlmdlgenlib/Buffer
      settings: SourceProductBaseCode=SL
  Saturation : Saturate  UpperLimit="fi(0,0,7,0,\"hex\",\"1f\")"  LowerLimit="fi(0,0,7,0,\"hex\",\"00\")"  SampleTime=0.258221781523715  OutDataTypeStr=fixdt(0, 7, 0)
  Saturation1 : Saturate  UpperLimit="fi(0,0,7,0,\"hex\",\"1f\")"  LowerLimit="fi(0,0,7,0,\"hex\",\"00\")"  SampleTime=0.258221781523715  OutDataTypeStr=fixdt(0, 7, 0)
  SignCorrected : Switch  Criteria=u2 ~= 0  Threshold=double(0)  OutDataTypeStr=fixdt(1, 17, 15)  SampleTime=0.258221781523715
  SignCorrected1 : Switch  Criteria=u2 ~= 0  Threshold=double(0)  OutDataTypeStr=fixdt(1, 17, 15)  SampleTime=0.258221781523715
  Switch : Switch  Criteria=u2 ~= 0  Threshold=double(0)  OutDataTypeStr=fixdt(0, 7, 0)  SampleTime=0.258221781523715
  Switch1 : Switch  Criteria=u2 ~= 0  Threshold=double(0)  OutDataTypeStr=fixdt(0, 7, 0)  SampleTime=0.258221781523715
  delayMatch : Delay  DelayLength=double(1)  InitialCondition=0  SampleTime=0.258221781523715
  delayMatch1 : Delay  DelayLength=double(1)  InitialCondition=0  SampleTime=0.258221781523715
  dtc : DataTypeConversion  OutDataTypeStr=uint8  SampleTime=0.258221781523715
  insig : DataTypeConversion  OutDataTypeStr=fixdt(0, 7, 7)  SampleTime=0.258221781523715
  insig1 : DataTypeConversion  OutDataTypeStr=fixdt(0, 7, 7)  SampleTime=0.258221781523715
  p25mA : Sum  Inputs=+-  AccumDataTypeStr=fixdt(1, 18, 17)  OutDataTypeStr=fixdt(1, 18, 17)  SampleTime=0.258221781523715
  p50mA : Sum  Inputs=+-  AccumDataTypeStr=fixdt(1, 19, 17)  OutDataTypeStr=fixdt(1, 19, 17)  SampleTime=0.258221781523715
  p75mA : Sum  Inputs=+-  AccumDataTypeStr=fixdt(1, 18, 17)  OutDataTypeStr=fixdt(1, 18, 17)  SampleTime=0.258221781523715
  pow2switch : Constant  OutDataTypeStr=boolean  SampleTime=0.258221781523715
  pow2switch1 : Constant  OutDataTypeStr=boolean  SampleTime=0.258221781523715
  x : Outport
  y : Outport  Port=2
  wires:
  dtc/1 -> RAMDelayBalance/1
  Amp25/1 -> QuadHandle1a/3
  Amp75/1 -> QuadHandle1b/1
  CastU16En1/1 -> CastU16En3/1
  CastU16En2/1 -> Switch/3, Saturation/1
  CastU16En3/1 -> CastU16En2/1
  GTEp75/1 -> QuadHandle1b/2, 1st or 4th Quad/2
  LTEp25/1 -> QuadHandle1a/2, 1st or 4th Quad/1
  LTEp50/1 -> QuadHandle2/2
  PipelineRegister/1 -> Positive/1, Negate/1
  Negate/1 -> SignCorrected/3
  Point25/1 -> p25mA/1, LTEp25/2, Amp25/2
  Point50/1 -> LTEp50/2
  Point75/1 -> p75mA/1, GTEp75/2, Amp75/2
  Positive/1 -> SignCorrected/1
  QuadHandle1a/1 -> QuadHandle2/1
  QuadHandle1b/1 -> QuadHandle2/3
  QuadHandle2/1 -> CastU16En1/1
  delayMatch1/1 -> SignCorrected/2
  Saturation/1 -> Switch/1
  SignCorrected/1 -> y/1
  Switch/1 -> Look-Up Table/1
  insig/1 -> p75mA/2, p25mA/2, LTEp50/1, LTEp25/1, GTEp75/1, Amp75/1, Amp25/1
  p25mA/1 -> QuadHandle1a/1
  p75mA/1 -> QuadHandle1b/3
  pow2switch/1 -> Switch/2
  Amp50/1 -> QuadHandle1/3
  CastU16En21/1 -> CastU16En4/1
  CastU16En31/1 -> Switch1/3, Saturation1/1
  CastU16En4/1 -> CastU16En31/1
  LTEp251/1 -> QuadHandle21/2
  LTEp501/1 -> QuadHandle1/2, RAMDelayBalance1/1
  PipelineRegister1/1 -> Positive1/1, Negate1/1
  Negate1/1 -> SignCorrected1/3
  Point251/1 -> LTEp251/2
  Point501/1 -> p50mA/1, LTEp501/2, Amp50/2
  Positive1/1 -> SignCorrected1/1
  QuadHandle1/1 -> p50mA/2, QuadHandle21/1, LTEp251/1
  QuadHandle21/1 -> CastU16En21/1
  delayMatch/1 -> SignCorrected1/2
  Saturation1/1 -> Switch1/1
  SignCorrected1/1 -> x/1
  Switch1/1 -> Look-Up Table1/1
  insig1/1 -> QuadHandle1/1, LTEp501/1, Amp50/1
  p50mA/1 -> QuadHandle21/3
  pow2switch1/1 -> Switch1/2
  1st or 4th Quad/1 -> dtc/1
  RAMDelayBalance1/1 -> delayMatch/1
  RAMDelayBalance/1 -> delayMatch1/1
  u/1 -> insig1/1, insig/1
  Look-Up Table/1 -> PipelineRegister/1
  Look-Up Table1/1 -> PipelineRegister1/1

== system gm_transmitter/tran_dut/bit_mapping/angle_selector ==
  input : Inport  OutDataTypeStr=fixdt(0, 3, 0)  PortDimensions=1  SampleTime=0.258221781523715
  angle_selector : MATLAB Function  TreatAsAtomicUnit=on
  phase : Outport  VectorParamsAs1DForOutWhenUnconnected=off
  wires:
  angle_selector/1(phase) -> phase/1
  input/1 -> angle_selector/1(input)

== system gm_transmitter/tran_dut/ldpc_encoder/MATLAB Function ==
  parity_in : Inport  OutDataTypeStr=fixdt(0, 1, 0)  PortDimensions=[16201]  SampleTime=2.06577425218972
  addresses : Inport  Port=2  OutDataTypeStr=uint16  PortDimensions=[1 12]  SampleTime=2.06577425218972
  input_bit : Inport  Port=3  OutDataTypeStr=boolean  PortDimensions=1  SampleTime=2.06577425218972
  MATLAB Function : MATLAB Function  TreatAsAtomicUnit=on
  parity_out : Outport  VectorParamsAs1DForOutWhenUnconnected=off
  wires:
  parity_in/1 -> MATLAB Function/1(parity_in)
  addresses/1 -> MATLAB Function/2(addresses)
  input_bit/1 -> MATLAB Function/3(input_bit)
  MATLAB Function/1(parity_out) -> parity_out/1

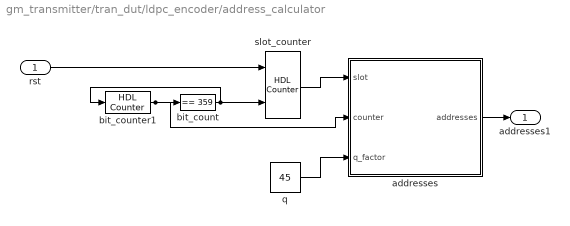
== system gm_transmitter/tran_dut/ldpc_encoder/address_calculator ==
  rst : Inport  OutDataTypeStr=boolean  PortDimensions=1  SampleTime=2.06577425218972
  addresses : Subsystem
  bit_count : simulink/Logic and Bit Operations/Compare To Constant  relop===  const=359  OutDataTypeStr=boolean
  bit_counter1 : hdlsllib/Sources/HDL Counter  CountType=Count limited  CountInit=0  CountStep=1  CountMax=359  CountFromType=Initial value  CountFrom=0  CountResetPort=on  CountLoadPort=off  CountEnbPort=off  CountDirPort=off  CountDataType=Unsigned  CountWordLen=9  CountFracLen=0  CountSampTime=1
  q : Constant  Value=45  OutDataTypeStr=uint8  SampleTime=-1
  slot_counter : hdlsllib/Sources/HDL Counter  CountType=Count limited  CountInit=1  CountStep=1  CountMax=135  CountFromType=Initial value  CountFrom=1  CountResetPort=on  CountLoadPort=off  CountEnbPort=on  CountDirPort=off  CountDataType=Unsigned  CountWordLen=8  CountFracLen=0  CountSampTime=1
  addresses1 : Outport
  wires:
  addresses/1(addresses) -> addresses1/1
  bit_count/1 -> slot_counter/2, bit_counter1/1
  bit_counter1/1 -> addresses/2(counter), bit_count/1
  q/1 -> addresses/3(q_factor)
  slot_counter/1 -> addresses/1(slot)
  rst/1 -> slot_counter/1

== system gm_transmitter/tran_dut/ldpc_encoder/p2s ==
  parallel_in : Inport  OutDataTypeStr=fixdt(0, 1, 0)  PortDimensions=[16201]  SampleTime=2.06577425218972
  enable : Inport  Port=2  OutDataTypeStr=boolean  PortDimensions=1  SampleTime=2.06577425218972
  p2s : MATLAB Function  TreatAsAtomicUnit=on  mask{input_length=16200}
  serial_out : Outport  VectorParamsAs1DForOutWhenUnconnected=off
  valid : Outport  Port=2
  wires:
  p2s/1(serial_out) -> serial_out/1
  p2s/2(valid) -> valid/1
  parallel_in/1 -> p2s/1(parallel_in)
  enable/1 -> p2s/2(enable)
